simulink model "nonlinear"  (R2021b)
settings: Solver=FixedStepAuto  StartTime=0.0  StopTime=RunTime  FixedStep=time_step  RelTol=1e-3
values from neighbouring files (symbols this model uses):
  g1 = (m_1 * c_1_0 + m_2 * l_1) * g    [compare_ourmodel_with_others.m]    (also in step4_0_linearize_operating_point.m = (m1 * c1 + m2 * l1) * g; step6_1_controller_feedback.m = (m1 * c1 + m2 * l1) * g)
  g2 = m_2 * c_2_0 * g    [compare_ourmodel_with_others.m]    (also in step4_0_linearize_operating_point.m = m2 * c2 * g; step6_1_controller_feedback.m = m2 * c2 * g)
  init_theta_1 = pi    (= 3.14159265359)    [compare_ourmodel_with_others.m]    (also in step2_whitebox_beam.m = theta_1(1); step2_whitebox_pend.m)
  init_theta_2 = 0    [compare_ourmodel_with_others.m]    (also in step2_whitebox_beam.m = theta_1(2); step2_whitebox_pend.m = -1.57079632679)
  P1 = m_1 * c_1_0 * c_1_0 + m_2 * l_1 * l_1 + I_1_0    [compare_ourmodel_with_others.m]    (also in step4_0_linearize_operating_point.m = m1 * c1 * c1 + m2 * l1 * l1 + I1; step6_1_controller_feedback.m = m1 * c1 * c1 + m2 * l1 * l1 + I1)
  P2 = m_2 * c_2_0 * c_2_0 + I_2_0    [compare_ourmodel_with_others.m]    (also in step4_0_linearize_operating_point.m = m2 * c2 * c2 + I2; step6_1_controller_feedback.m = m2 * c2 * c2 + I2)
  P3 = m_2 * l_1 * c_2_0    [compare_ourmodel_with_others.m]    (also in step4_0_linearize_operating_point.m = m2 * l1 * c2; step6_1_controller_feedback.m = m2 * l1 * c2)
  params = [9.81, 0.1, 0.1, 0.125, 0.0487, -0.0286, 0.0624, 0.0169, 6.81e-5, 6.9742, 2.89e-05, 46.1069, 0.0308]    [compare_ourmodel_with_others.m]    (also in costfun.m = x; step2_whitebox_pend.m = x; step4_linearized_system.mat = [9.81 0.1 0.1 0.125 0.046955 -0.032 0.04609 0.0088 9.8e-05 6)
settings Model: Creator=basti  LastModifiedBy=lyitingli

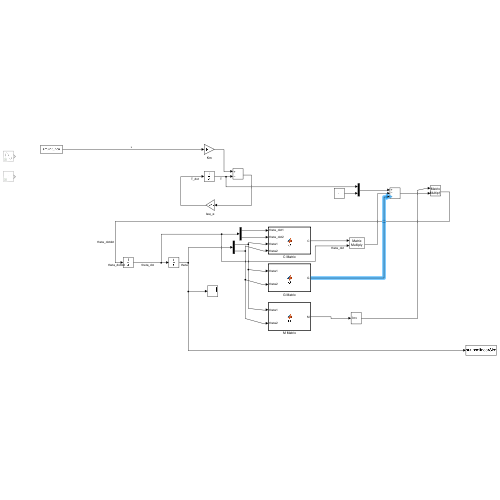
[thumbnail: Simulink's stored preview of the top-level diagram]
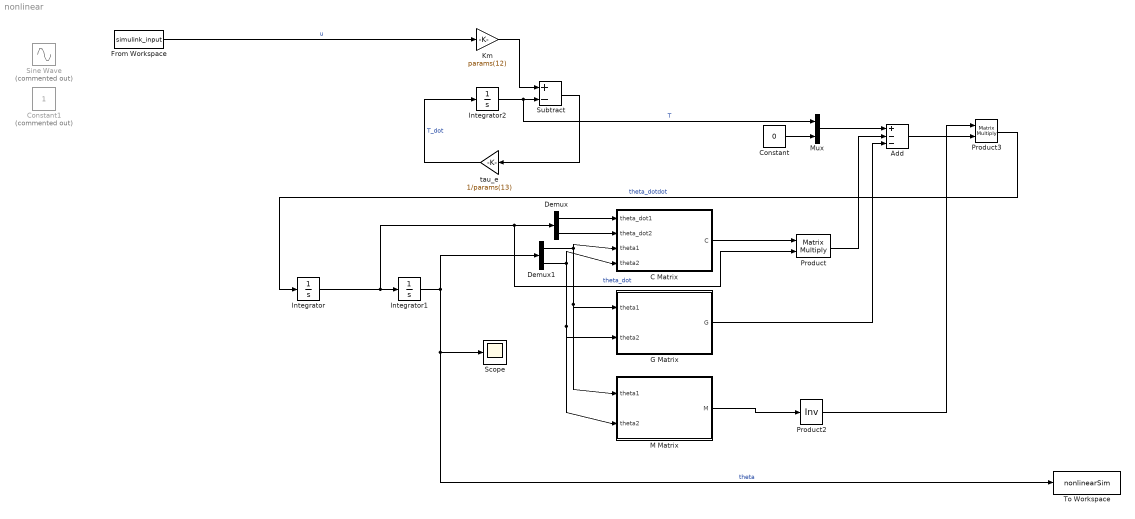
== system nonlinear ==
  Add : Sum  Inputs=+--
  C Matrix : MATLAB Function  TreatAsAtomicUnit=on
  Constant : Constant  Value=0
  Constant1 : Constant  Commented=on
  Demux : Demux  Outputs=2
  Demux1 : Demux  Outputs=2
  From Workspace : FromWorkspace  SampleTime=-1
  G Matrix : MATLAB Function  TreatAsAtomicUnit=on
  Integrator : Integrator
  Integrator1 : Integrator  InitialCondition=[init_theta_1, init_theta_2]
  Integrator2 : Integrator
  Km : Gain  Gain=params(12)
  M Matrix : MATLAB Function  TreatAsAtomicUnit=on
  Mux : Mux  Inputs=2
  Product : Product  Inputs=**  Multiplication=Matrix(*)
  Product2 : Product  Inputs=/  Multiplication=Matrix(*)
  Product3 : Product  Inputs=**  Multiplication=Matrix(*)
  Scope : Scope
  Sine Wave : Sin  Commented=on  Amplitude=4  Frequency=4  SampleTime=0
  Subtract : Sum  Inputs=+-
  To Workspace : ToWorkspace  VariableName=nonlinearSim  SampleTime=0.001
  tau_e : Gain  Gain=1/params(13)
  wires:
  Integrator/1 -> Product/2, Demux/1, Integrator1/1  "theta_dot"
  Product3/1 -> Integrator/1  "theta_dotdot"
  Integrator1/1 -> To Workspace/1, Scope/1, Demux1/1  "theta"
  C Matrix/1(C) -> Product/1
  tau_e/1 -> Integrator2/1  "T_dot"
  Integrator2/1 -> Mux/1, Subtract/2  "T"
  From Workspace/1 -> Km/1  "u"
  Km/1 -> Subtract/1
  Subtract/1 -> tau_e/1
  Product/1 -> Add/2
  G Matrix/1(G) -> Add/3
  M Matrix/1(M) -> Product2/1
  Product2/1 -> Product3/1
  Add/1 -> Product3/2
  Constant/1 -> Mux/2
  Mux/1 -> Add/1
  Demux1/1 -> C Matrix/3(theta1), M Matrix/1(theta1), G Matrix/1(theta1)
  Demux1/2 -> C Matrix/4(theta2), M Matrix/2(theta2), G Matrix/2(theta2)
  Demux/1 -> C Matrix/1(theta_dot1)
  Demux/2 -> C Matrix/2(theta_dot2)

== matlab function nonlinear/C Matrix ==
  data: theta_dot1 input; theta_dot2 input; theta1 input; theta2 input; C output; params parameter; P3 parameter
function C = C(theta_dot1, theta_dot2, theta1, theta2, params, P3)
c00 = params(10)-P3*theta_dot2*sin(theta2);
c01 = -P3*(theta_dot1+theta_dot2)*sin(theta2);
c10 = P3*theta_dot1*sin(theta2);
c11 = params(11);
C = [c00 c01; c10 c11];

== matlab function nonlinear/G Matrix ==
  data: theta1 input; theta2 input; G output; g1 parameter; g2 parameter
function G = G(theta1, theta2, g1, g2)
g00 = -g1*sin(theta1)-g2*sin(theta1+theta2);
g01 = -g2*sin(theta1+theta2);
G = [g00 g01];

== matlab function nonlinear/M Matrix ==
  data: theta1 input; theta2 input; M output; P1 parameter; P2 parameter; P3 parameter
function M = M(theta1, theta2, P1, P2, P3)
m00 = P1+P2+2*P3*cos(theta2);
m01 = P2+P3*cos(theta2);
m10 = m01;
m11 = P2;
M = [m00 m01; m10 m11];
